simulink model "spring_mass_damper_system"  (R2022b)
settings: Solver=FixedStepAuto  StartTime=0.0  StopTime=Tf  FixedStep=dt  RelTol=1e-3
values from neighbouring files (symbols this model uses):
  c = 1    [slx_main.m]
  k = 10    [slx_main.m]
  m = 1    [slx_main.m]
  v0 = 0    [slx_main.m]
  x0 = 1    [slx_main.m]
settings Model: Creator=murayama  LastModifiedBy=murayama
settings DataIOCC: ReturnWorkspaceOutputs=off

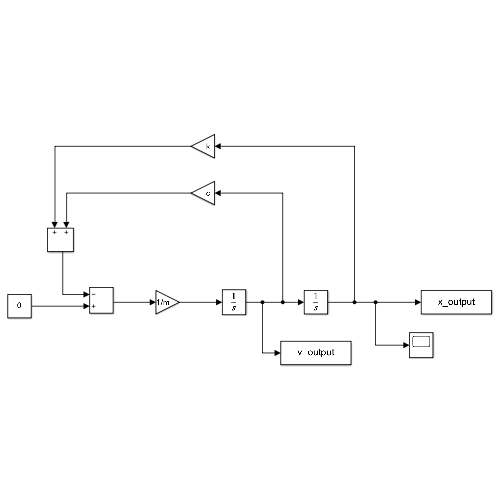
[thumbnail: Simulink's stored preview of the top-level diagram]
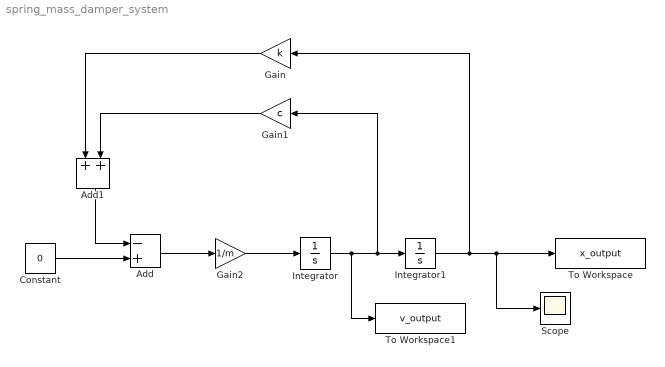
== system spring_mass_damper_system ==
  Add : Sum  Inputs=-+
  Add1 : Sum
  Constant : Constant  Value=0
  Gain : Gain  Gain=k
  Gain1 : Gain  Gain=c
  Gain2 : Gain  Gain=1/m
  Integrator : Integrator  InitialCondition=v0
  Integrator1 : Integrator  InitialCondition=x0
  Scope : Scope
  To Workspace : ToWorkspace  VariableName=x_output  SaveFormat=Timeseries  SampleTime=-1
  To Workspace1 : ToWorkspace  VariableName=v_output  SaveFormat=Timeseries  SampleTime=-1
  wires:
  Gain2/1 -> Integrator/1
  Integrator/1 -> To Workspace1/1, Gain1/1, Integrator1/1
  Add/1 -> Gain2/1
  Integrator1/1 -> Gain/1, To Workspace/1, Scope/1
  Gain1/1 -> Add1/2
  Add1/1 -> Add/1
  Gain/1 -> Add1/1
  Constant/1 -> Add/2
